simulink model "myprojecttwo"  (R2023b)
settings: Solver=VariableStepAuto  StartTime=0.0  StopTime=0.01  RelTol=1e-3
libraries: spsSeriesRLCBranchLib x3, spsCurrentMeasurementLib x3, spsVoltageMeasurementLib x2, spsDCVoltageSourceLib x1, spsDiodeLib x1, spsMosfetLib x1, sps_lib x1
settings Model: Creator=mrrid  LastModifiedBy=mrrid

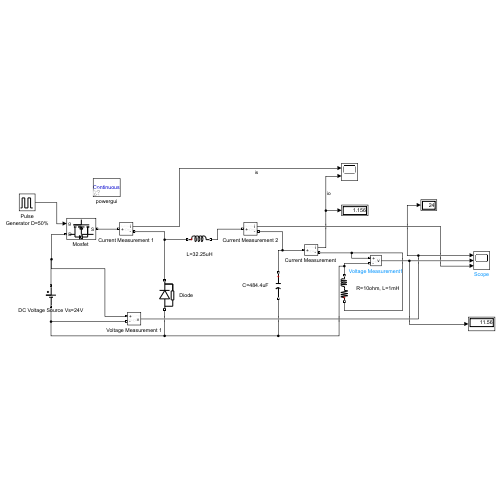
[thumbnail: Simulink's stored preview of the top-level diagram]
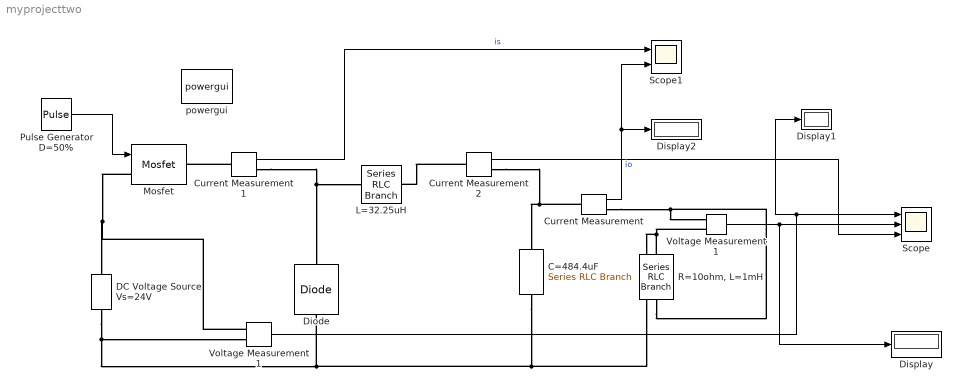
== system myprojecttwo ==
  " L=32.25uH" : spsSeriesRLCBranchLib/Series RLC Branch  LConnTagsString=__new0  RConnTagsString=__new0  BranchType=L  Resistance=1  Inductance=32.25e-6  SetiL0=off  InitialCurrent=0  Capacitance=1e-6  Setx0=off  InitialVoltage=0  Measurements=None
  C=484.4uF : spsSeriesRLCBranchLib/Series RLC Branch  LConnTagsString=__new0  RConnTagsString=__new0  BranchType=C  Resistance=1  Inductance=1e-3  SetiL0=off  InitialCurrent=0  Capacitance=484.4e-6  Setx0=off  InitialVoltage=0  Measurements=None
  "Current Measurement " : spsCurrentMeasurementLib/Current Measurement  PhasorSimulation=off  OutputType=Complex  PSBequivalent=0
  Current Measurement 1 : spsCurrentMeasurementLib/Current Measurement  PhasorSimulation=off  OutputType=Complex  PSBequivalent=0
  Current Measurement 2 : spsCurrentMeasurementLib/Current Measurement  PhasorSimulation=off  OutputType=Complex  PSBequivalent=0
  DC Voltage Source Vs=24V : spsDCVoltageSourceLib/DC Voltage Source  Amplitude=24  Measurements=Voltage
  "Diode " : spsDiodeLib/Diode  Ron=0.001  Lon=0  Vf=0.8  IC=0  UseSnubber=0  Rs=500  Cs=250e-9  Measurements=off
  Display : Display
  Display1 : Display
  Display2 : Display
  "Mosfet " : spsMosfetLib/Mosfet  Ron=0.1  Lon=0  Rd=0.01  Vfd=0  IC=0  Rs=1e5  Cs=inf  Measurements=off
  Pulse Generator D=50% : DiscretePulseGenerator  PulseType=Time based  Amplitude=10  Period=0.000005  PulseWidth=50
  "R=10ohm, L=1mH" : spsSeriesRLCBranchLib/Series RLC Branch  LConnTagsString=__new0  RConnTagsString=__new0  BranchType=RL  Resistance=10  Inductance=1e-3  SetiL0=off  InitialCurrent=0  Capacitance=1e-6  Setx0=off  InitialVoltage=0  Measurements=None
  Scope : Scope  NumInputPorts=3
  Scope1 : Scope  NumInputPorts=2
  Voltage Measurement 1 : spsVoltageMeasurementLib/Voltage Measurement  PhasorSimulation=off  OutputType=Complex  PSBequivalent=0
  Voltage Measurement1 : spsVoltageMeasurementLib/Voltage Measurement  PhasorSimulation=off  OutputType=Complex  PSBequivalent=0
  powergui : sps_lib/powergui  Priority=1  SimulationMode=Continuous  SampleTime=50e-6  frequency=60  Iterations=50  frequencyindice=0  Pbase=100e6  ErrMax=1e-4  UnitsV=kV  UnitsW=MW  buscounter=0  FunctionMessages=off  echomessages=off  EnableUseOfTLC=off  CurrentSourceSwitches=off  DisableSnubberDevices=off  DisableRonSwitches=off  DisableVfSwitches=off  DisplayEquations=off  AutomaticDiscreteSolvers=off  SolverType=Tustin/Backward Euler (TBE)  Interpol=off  ExternalGateDelay=off  methode=off  Ts=100  x0status=blocks  SPID=on  SwTol=0  HookPort=off  NonlinearTolerance=1e-4  nMaxIteration=100  ContinueOnMaxIteration=off  RestoreLinks=warning  ResistiveCurrentMeasurement=off  Frange=[0:2:500]  Ylog=off  Xlog=on  ShowGrid=off  save=off  variable=ZData  structure=0  ZoomFFT=off  StartTime=0.0  cycles=1  DisplayStyle=1  fundamental=60  FreqAxis=off  MaxFrequency=1000  frequencyindicesteady=1  RmsSteady=1  display=off
  wires:
  Pulse Generator D=50%/1 -> "Mosfet "/1
  Current Measurement 1/1 -> Scope1/1  "is"
  Current Measurement 2/1 -> Scope/3
  Voltage Measurement1/1 -> Display/1, Scope/2
  Voltage Measurement 1/1 -> Display1/1, Scope/1
  "Current Measurement "/1 -> Display2/1, Scope1/2  "io"
  connections:
  "Mosfet "/LConn1 -- Voltage Measurement 1/LConn1 -- DC Voltage Source Vs=24V/RConn1
  DC Voltage Source Vs=24V/LConn1 -- Voltage Measurement 1/LConn2 -- "R=10ohm, L=1mH"/RConn1 -- Voltage Measurement1/LConn2 -- C=484.4uF/RConn1 -- "Diode "/LConn1
  Current Measurement 1/LConn1 -- "Mosfet "/RConn1
  Current Measurement 1/RConn1 -- " L=32.25uH"/LConn1 -- "Diode "/RConn1
  Current Measurement 2/LConn1 -- " L=32.25uH"/RConn1
  Current Measurement 2/RConn1 -- "Current Measurement "/LConn1 -- C=484.4uF/LConn1
  "Current Measurement "/RConn1 -- "R=10ohm, L=1mH"/LConn1 -- Voltage Measurement1/LConn1
